simulink model "Temperature_Control_System"  (R2019a)
settings: Solver=FixedStepAuto  StartTime=0.0  StopTime=10  FixedStep=0.0001  RelTol=1e-3
libraries: fl_lib x29, nesl_utility x10, fl_ps_legacy_lib x3, ee_lib x3, simulink x1
settings Model: Creator=CXJ889  LastModifiedBy=willi

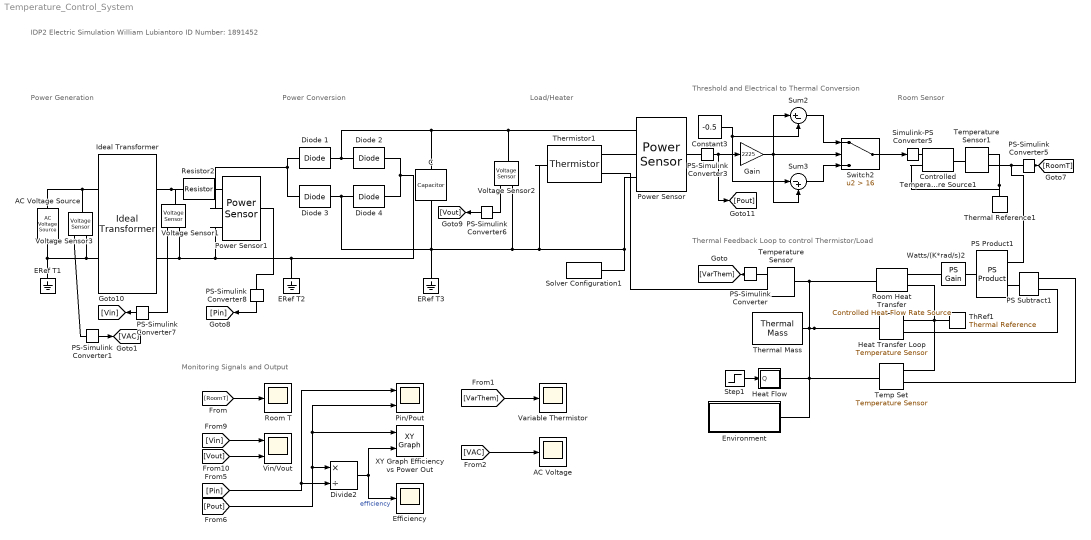
== system Temperature_Control_System ==
  note: IDP2 Electric Simulation
      | William Lubiantoro
      | ID Number: 1891452
  note: Thermal Feedback Loop to control Thermistor/Load
  note: Room Sensor
  note: Power Generation
  note: Load/Heater
  note: Threshold and Electrical to Thermal Conversion
  note: Power Conversion
  note: Monitoring Signals and Output
  AC Voltage Source : fl_lib/Electrical/Electrical Sources/AC Voltage Source  amp=220 V  shift=0 deg  frequency=50 Hz  omega=0 rad/s
  AC Voltage : Scope
  C : fl_lib/Electrical/Electrical Elements/Capacitor  c=1000e-06 F  r=1e-06 Ohm  g=0 1/Ohm  i_specify=off  i_priority=High  i=0 A  i_nominal_specify=off  i_nominal_unit=A  i_nominal_value=1  v_specify=off  v_priority=High  v=0 V  v_nominal_specify=off  v_nominal_unit=V  v_nominal_value=1  vc_specify=on  vc_priority=High  vc=0 V  vc_nominal_specify=off  vc_nominal_unit=V  vc_nominal_value=1
  Constant3 : Constant  Value=-0.5
  Controlled Temperature Source1 : fl_lib/Thermal/Thermal Sources/Controlled Temperature Source
      settings: SourceProductName=Simscape
  Diode {1..4} (4 alike) : fl_lib/Electrical/Electrical Elements/Diode  Vf=0.6 V  Ron=0.3 Ohm  Goff=1e-08 1/Ohm  i_specify=off  i_priority=High  i=0 A  i_nominal_specify=off  i_nominal_unit=A  i_nominal_value=1  v_specify=off  v_priority=High  v=0 V  v_nominal_specify=off  v_nominal_unit=V  v_nominal_value=1
  Divide2 : Product  Inputs=*/
  ERef T1 : fl_lib/Electrical/Electrical Elements/Electrical Reference
  ERef T2 : fl_lib/Electrical/Electrical Elements/Electrical Reference
  ERef T3 : fl_lib/Electrical/Electrical Elements/Electrical Reference
  "Efficiency " : Scope
  "Environment " : Subsystem
      mask Display: disp('Set Room Temp')
  Gain : Gain  Gain=2225
  Heat Flow : Subsystem
  "Heat Transfer Loop " : fl_lib/Thermal/Thermal Sensors/Temperature Sensor
  Ideal Transformer : fl_lib/Electrical/Electrical Elements/Ideal Transformer  n=14  i1_specify=off  i1_priority=High  i1=0 A  i1_nominal_specify=off  i1_nominal_unit=A  i1_nominal_value=1  v1_specify=on  v1_priority=High  v1=220 V  v1_nominal_specify=off  v1_nominal_unit=V  v1_nominal_value=1  i2_specify=off  i2_priority=High  i2=0 A  i2_nominal_specify=off  i2_nominal_unit=A  i2_nominal_value=1  v2_specify=on  v2_priority=High  v2=12 V  v2_nominal_specify=off  v2_nominal_unit=V  v2_nominal_value=1
      settings: SourceProductName=Simscape  SourceProductBaseCode=SS
  PS Product1 : fl_ps_legacy_lib/Legacy Physical Signals/Functions/PS Product
      settings: SourceProductName=Simscape  SourceProductBaseCode=SS
  PS Subtract1 : fl_ps_legacy_lib/Legacy Physical Signals/Functions/PS Subtract
      settings: SourceProductName=Simscape  SourceProductBaseCode=SS
  PS-Simulink Converter : nesl_utility/PS-Simulink Converter  PhysicalDomain=network_engine_domain  SubClassName=ps_output  LeftPortType=input  RightPortType=output  PseudoPeriodic=off  Frequencies=[]  Unit=degC  AffineConversion=off
  PS-Simulink Converter{1,6..8} (4 alike) : nesl_utility/PS-Simulink Converter  PhysicalDomain=network_engine_domain  SubClassName=ps_output  LeftPortType=input  RightPortType=output  PseudoPeriodic=off  Frequencies=[]  Unit=1  AffineConversion=off
  PS-Simulink Converter3 : nesl_utility/PS-Simulink Converter  PhysicalDomain=network_engine_domain  SubClassName=ps_output  LeftPortType=input  RightPortType=output  PseudoPeriodic=off  Frequencies=[]  Unit=J/s  AffineConversion=off
  PS-Simulink Converter5 : nesl_utility/PS-Simulink Converter  PhysicalDomain=network_engine_domain  SubClassName=ps_output  LeftPortType=input  RightPortType=output  PseudoPeriodic=off  Frequencies=[]  Unit=degC  AffineConversion=off
  "Pin/Pout " : Scope  NumInputPorts=2
  Power Sensor : ee_lib/Sensors & Transducers/Power Sensor  measurement_type=1  averaging_period=1e-4 s
      settings: SourceProductName=Simscape Electrical  SourceProductBaseCode=PS
  Power Sensor1 : ee_lib/Sensors & Transducers/Power Sensor  measurement_type=1  averaging_period=1e-4 s
      settings: SourceProductName=Simscape Electrical  SourceProductBaseCode=PS
  Resistor2 : fl_lib/Electrical/Electrical Elements/Resistor  R=1250 Ohm  i_specify=off  i_priority=None  i=0 A  i_nominal_specify=off  i_nominal_unit=A  i_nominal_value=1  v_specify=off  v_priority=None  v=0 V  v_nominal_specify=off  v_nominal_unit=V  v_nominal_value=1
  "Room Heat Transfer " : fl_lib/Thermal/Thermal Sources/Controlled Heat Flow Rate Source
      settings: SourceProductName=Simscape
  "Room T " : Scope
  Simulink-PS Converter5 : nesl_utility/Simulink-PS Converter  PhysicalDomain=network_engine_domain  SubClassName=ps_input  LeftPortType=input  RightPortType=output  PseudoPeriodic=off  Frequencies=[]  NoiseDistribution=none  NoiseParameters=[]  Unit=degC  AffineConversion=off  FilteringAndDerivatives=provide  SimscapeFilterOrder=1  InputFilterTimeConstant=0.001  UdotUserProvided=0
  Solver Configuration1 : nesl_utility/Solver Configuration  PhysicalDomain=network_engine_domain  SubClassName=solver  LeftPortType=input  RightPortType=generic  Tones=[]  Harmonics=[]  SimulateNoise=off  Profile=off  UseLocalSampling=off  EnableSwitchedLinearOptims=on  FrequencyDomain=off  UseCCode=off  RelTol=0.001  AbsTol=1e-06  MinStep=1e-09  ToWorkspace=off  RevertToSquareIcSolve=off  NumHomotopyIterations=100  PhasorMode=off  PhasorModeNumHarmonics=1  DoDC=off  ResidualTolerance=1e-6  UseLocalSolver=off  LocalSolverChoice=NE_BACKWARD_EULER_ADVANCER  LocalSolverSampleTime=.001  DoFixedCost=off  MaxNonlinIter=3  MaxModeIter=2  LinearAlgebra=auto  EquationFormulation=NE_TIME_EF  DelaysMemoryBudget=1024  AutomaticFiltering=on  FilteringTimeConstant=0.001  PartitionStorageMethod=AS_NEEDED  PartitionMemoryBudget=1024  PartitionMethod=FAST
  Step1 : Step  Time=100  Before=10  After=20  SampleTime=0
      settings: AttributesFormatString=%<Time> sec
  Sum2 : Sum  Inputs=|+-
  Sum3 : Sum  Inputs=|-+
  Switch2 : Switch  Criteria=u2 > Threshold  Threshold=16
  "Temp Set " : fl_lib/Thermal/Thermal Sensors/Temperature Sensor
  Temperature Sensor : fl_lib/Thermal/Thermal Sensors/Temperature Sensor
  Temperature Sensor1 : fl_lib/Thermal/Thermal Sensors/Temperature Sensor
  ThRef1 : fl_lib/Thermal/Thermal Elements/Thermal Reference
  Thermal Mass : fl_lib/Thermal/Thermal Elements/Thermal Mass  mass=0.1 kg  sp_heat=100 J/kg/K  T_specify=on  T_priority=High  T=298.15 K  T_nominal_specify=off  T_nominal_unit=K  T_nominal_value=1  Q_specify=off  Q_priority=High  Q=0 J/s  Q_nominal_specify=off  Q_nominal_unit=J/s  Q_nominal_value=1
  Thermal Reference1 : fl_lib/Thermal/Thermal Elements/Thermal Reference
  Thermistor1 : ee_lib/Sensors & Transducers/Thermistor  R0=1000 Ohm  Bparam=1500 K  T0=273+16 K  tc=5.0 s  K_d=0.75e-3 W/K  T_specify=off  T_priority=High  T=298.15 K  T_nominal_specify=off  T_nominal_unit=K  T_nominal_value=1
      settings: SourceProductName=Simscape Electrical  SourceProductBaseCode=PS
  "Variable Thermistor " : Scope
  "Vin/Vout " : Scope  NumInputPorts=2
  Voltage Sensor1 : fl_lib/Electrical/Electrical Sensors/Voltage Sensor
  Voltage Sensor2 : fl_lib/Electrical/Electrical Sensors/Voltage Sensor
  Voltage Sensor3 : fl_lib/Electrical/Electrical Sensors/Voltage Sensor
  Watts/(K*rad/s)2 : fl_ps_legacy_lib/Legacy Physical Signals/Functions/PS Gain  gain=0.03
      settings: SourceProductName=Simscape
  "XY Graph Efficiency vs Power Out " : simulink/Sinks/XY Graph  xmin=-10  xmax=10  ymin=-10  ymax=10  st=50
  wires:
  [Pout] -> Divide2/1, "XY Graph Efficiency vs Power Out "/1, "Pin/Pout "/2
  Divide2/1 -> "Efficiency "/1, "XY Graph Efficiency vs Power Out "/2  "efficiency"
  PS-Simulink Converter6/1 -> [Vout]
  Sum2/1 -> Switch2/1
  Gain/1 -> Switch2/2, Sum3/2, Sum2/1
  Sum3/1 -> Switch2/3
  PS-Simulink Converter5/1 -> [RoomT]
  [RoomT] -> "Room T "/1
  PS-Simulink Converter8/1 -> [Pin]
  Switch2/1 -> Simulink-PS Converter5/1
  [Vout] -> "Vin/Vout "/2
  [Pin] -> Divide2/2, "Pin/Pout "/1
  PS-Simulink Converter7/1 -> [Vin]
  PS-Simulink Converter3/1 -> [Pout], Gain/1
  Constant3/1 -> Sum3/1, Sum2/2
  Step1/1 -> Heat Flow/1(Q)
  [Vin] -> "Vin/Vout "/1
  PS-Simulink Converter/1 -> [VarThem]
  [VarThem] -> "Variable Thermistor "/1
  PS-Simulink Converter1/1 -> [VAC]
  [VAC] -> AC Voltage/1
  connections:
  ERef T2/LConn1 -- Diode 4/RConn1 -- Diode 2/LConn1 -- Ideal Transformer/RConn2 -- Voltage Sensor1/RConn2 -- Power Sensor1/LConn3
  Temperature Sensor1/RConn1 -- Controlled Temperature Source1/RConn2 -- Thermal Reference1/LConn1
  Voltage Sensor2/RConn2 -- Diode 4/LConn1 -- Diode 3/LConn1 -- ERef T3/LConn1 -- C/RConn1 -- Thermistor1/RConn1 -- Power Sensor/LConn3 -- Solver Configuration1/RConn1
  ERef T1/LConn1 -- Voltage Sensor3/RConn2 -- Ideal Transformer/LConn2 -- AC Voltage Source/RConn1
  PS-Simulink Converter5/LConn1 -- PS Product1/LConn1 -- Temperature Sensor1/RConn2
  Power Sensor/LConn1 -- Diode 1/RConn1 -- Diode 2/RConn1 -- C/LConn1 -- Voltage Sensor2/LConn1
  "Room Heat Transfer "/LConn1 -- Temperature Sensor/LConn1 -- Thermal Mass/LConn1 -- "Heat Transfer Loop "/LConn1 -- Heat Flow/RConn1 -- "Environment "/LConn1 -- "Temp Set "/LConn1
  "Heat Transfer Loop "/RConn1 -- "Room Heat Transfer "/RConn2 -- ThRef1/LConn1 -- "Temp Set "/RConn1
  Diode 1/LConn1 -- Diode 3/RConn1 -- Power Sensor1/LConn2
  Voltage Sensor1/LConn1 -- Ideal Transformer/RConn1 -- Resistor2/LConn1
  Watts/(K*rad/s)2/LConn1 -- PS Product1/RConn1
  Voltage Sensor2/RConn1 -- PS-Simulink Converter6/LConn1
  Voltage Sensor1/RConn1 -- PS-Simulink Converter7/LConn1
  PS-Simulink Converter3/LConn1 -- Power Sensor/RConn1
  Controlled Temperature Source1/LConn1 -- Temperature Sensor1/LConn1
  Simulink-PS Converter5/RConn1 -- Controlled Temperature Source1/RConn1
  Ideal Transformer/LConn1 -- Voltage Sensor3/LConn1 -- AC Voltage Source/LConn1
  PS Product1/LConn2 -- PS Subtract1/RConn1
  "Room Heat Transfer "/RConn1 -- Watts/(K*rad/s)2/RConn1
  "Temp Set "/RConn2 -- PS Subtract1/LConn1
  PS-Simulink Converter8/LConn1 -- Power Sensor1/RConn1
  Power Sensor1/LConn1 -- Resistor2/RConn1
  Thermistor1/LConn2 -- Power Sensor/LConn2
  "Heat Transfer Loop "/RConn2 -- PS Subtract1/LConn2
  Temperature Sensor/RConn1 -- Thermistor1/LConn1
  Temperature Sensor/RConn2 -- PS-Simulink Converter/LConn1
  Voltage Sensor3/RConn1 -- PS-Simulink Converter1/LConn1

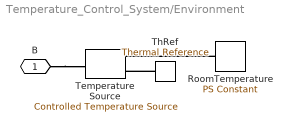
== system Temperature_Control_System/Environment  ==
  RoomTemperature : fl_lib/Physical Signals/Sources/PS Constant  constant=273.15+16
  Temperature Source : fl_lib/Thermal/Thermal Sources/Controlled Temperature Source
      settings: SourceProductName=Simscape
  ThRef : fl_lib/Thermal/Thermal Elements/Thermal Reference
  B : PMIOPort  Side=Left
  connections:
  RoomTemperature/RConn1 -- Temperature Source/RConn1
  ThRef/LConn1 -- Temperature Source/RConn2
  B/RConn1 -- Temperature Source/LConn1

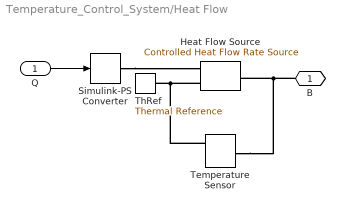
== system Temperature_Control_System/Heat Flow ==
  Q : Inport
  Heat Flow Source : fl_lib/Thermal/Thermal Sources/Controlled Heat Flow Rate Source
      settings: SourceProductName=Simscape
  Simulink-PS Converter : nesl_utility/Simulink-PS Converter  PhysicalDomain=network_engine_domain  SubClassName=ps_input  LeftPortType=input  RightPortType=output  PseudoPeriodic=off  Frequencies=[]  NoiseDistribution=none  NoiseParameters=[]  Unit=1  AffineConversion=off  FilteringAndDerivatives=zero  SimscapeFilterOrder=1  InputFilterTimeConstant=.001  UdotUserProvided=0
  Temperature Sensor : fl_lib/Thermal/Thermal Sensors/Temperature Sensor
  ThRef : fl_lib/Thermal/Thermal Elements/Thermal Reference
  B : PMIOPort  Side=Right
  wires:
  Q/1 -> Simulink-PS Converter/1
  connections:
  Heat Flow Source/RConn2 -- Temperature Sensor/RConn1 -- ThRef/LConn1
  Simulink-PS Converter/RConn1 -- Heat Flow Source/RConn1
  B/RConn1 -- Temperature Sensor/LConn1 -- Heat Flow Source/LConn1
